simulink model "Model_TAGGED"  (R2022b)
settings: Solver=FixedStepDiscrete  StartTime=0.0  StopTime=100  RelTol=1e-3  EnableMultiTasking=on
InitFcn:
  | % Initialize model
  | ModelSettings=BTConfig.GetModelSettings();
  | 
  | ModelSettings.Validate();
  | 
  | ModelInit;
  | 
  | 
  | % load library data
  | GainLibrary_data;
StartFcn:
  | % make sure all the simulated RTC requests are found
  | %RTC_SIM_OBJ.ValidateREQs();
undefined symbols (not defined in the file or in its folder): MedusaConfig, sys_defs
libraries: FeaturePath x17, RTC x8, SampleRateConverterBtc x4, dspindex x3, EdgePorts x2, medusa5h1_stereo x2, FadeRamper x2, MuteRamper x2, SleepingBeauty x2, ToneBtc x2, dspsrcs4 x2, RouterBtc x1
(part 1 of 2)
settings Model: Creator=kl13806  LastModifiedBy=mp55777
settings SolverCC: AlgebraicLoopSolver=TrustRegion  AutoInsertRateTranBlk=on
settings OptimizationCC: DefaultParameterBehavior=Inlined  DefaultUnderspecifiedDataType=single  ZeroExternalMemoryAtStartup=off  ZeroInternalMemoryAtStartup=off  MaxStackSize=2048  DifferentSizesBufferReuse=on  EfficientTunableParamExpr=on
settings DebuggingCC: InheritedTsInSrcMsg=none  MultiTaskDSMMsg=none  MultiTaskRateTransMsg=warning  ParameterPrecisionLossMsg=none  ParameterTunabilityLossMsg=error  UnconnectedInputMsg=warning  UnconnectedOutputMsg=warning  UnconnectedLineMsg=warning  BusObjectLabelMismatch=none  UnknownTsInhSupMsg=none  SFUnexpectedBacktrackingDiag=warning  SFNoUnconditionalDefaultTransitionDiag=warning  SFExecutionAtInitializationDiag=none  SFMachineParentedDataDiag=warning  ArithmeticOperatorsInVariantConditions=warning
settings HardwareCC: ProdBitPerDouble=32  ProdBitPerPointer=32  ProdBitPerSizeT=32  ProdBitPerPtrDiffT=32  ProdLargestAtomicInteger=Long  ProdLargestAtomicFloat=Double  ProdWordSize=32  ProdHWDeviceType=Qualcomm->Hexagon  TargetBitPerPointer=64  TargetBitPerSizeT=64  TargetBitPerPtrDiffT=64  TargetLargestAtomicInteger=Integer  TargetLongLongMode=on  TargetIntDivRoundTo=Zero  TargetEndianess=LittleEndian  TargetWordSize=64  TargetHWDeviceType=MATLAB Host  ProdEqTarget=off
settings ModelReferenceCC: EnableRefExpFcnMdlSchedulingChecks=on
settings SFSimCC: SimUseLocalCustomCode=off  MATLABDynamicMemAlloc=off  CustomCodeUndefinedFunction=UseInterfaceOnly
settings RTWCC: Description=Embedded Coder (host-based shared library target)  SystemTargetFile=ert_shrlib.tlc  GenCodeOnly=on  TemplateMakefile=ert_default_tmf  GenerateReport=on  RetainRTWFile=on  RTWUseLocalCustomCode=off  BuildConfiguration=Faster Runs  IncludeHyperlinkInReport=on  GenerateTraceInfo=on  GenerateTraceReport=on  GenerateTraceReportSl=on  GenerateTraceReportSf=on  GenerateTraceReportEml=on  GenerateCodeMetricsReport=on  GenerateCodeReplacementReport=on
settings CodeAppCC: ForceParamTrailComments=on  IgnoreCustomStorageClasses=off  MaxIdLength=61  OperatorAnnotations=on  SimulinkDataObjDesc=on  SFDataObjDesc=on  MATLABFcnDesc=on  InsertBlockDesc=on  StateflowObjectComments=on  MATLABSourceComments=on
settings STFCustomTargetCC: TargetLangStandard=C99 (ISO)  CodeReplacementLibrary=Qualcomm Hexagon DSP code replacement library,ARM Neon V7/V8 code replacement library  ParMdlRefBuildCompliant=on  CompOptLevelCompliant=on  CombineOutputUpdateFcns=on  ERTCustomFileBanners=on  SupportNonFinite=off  SupportContinuousTime=off  SupportNonInlinedSFcns=off  RemoveResetFunc=on  SupportVariableSizeSignals=on  MATLABClassNameForMDSCustomization=Simulink.SoftwareTarget.ERTCustomization  ModelStepFunctionPrototypeControlCompliant=on  UseToolchainInfoCompliant=on  SystemTargetFile=ert_shrlib.tlc
settings ERTTargetCC: TargetLangStandard=C99 (ISO)  CodeReplacementLibrary=Qualcomm Hexagon DSP code replacement library,ARM Neon V7/V8 code replacement library  MultiwordLength=2048  ConcurrentExecutionCompliant=off  SupportNonFinite=off  SupportVariableSizeSignals=on  CPPClassGenCompliant=off  InlinedParameterPlacement=NonHierarchical  ERTCustomFileTemplate=example_file_process.tlc  IndentStyle=Allman  IndentSize=4
settings ConfigComp: CovMetricSettings=dw  CovSaveCumulativeToWorkspaceVar=on  CovSaveSingleToWorkspaceVar=on  CovExternalEMLEnable=off

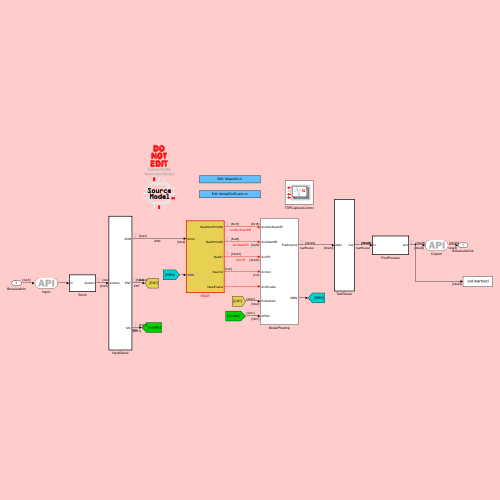
[thumbnail: Simulink's stored preview of the top-level diagram]
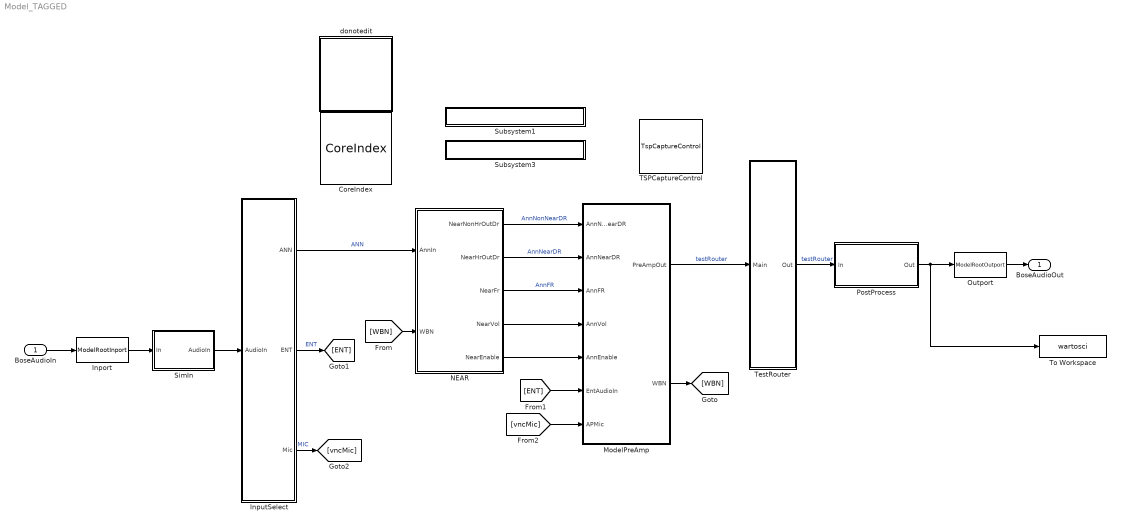
== system Model_TAGGED ==
  BoseAudioIn : Inport  OutDataTypeStr=single  PortDimensions=[ModelSettings.ModelFrameSize (ModelSettings.NumInputAudioChannels + ModelSettings.NumInputMicChannels)]  SampleTime=1/sys_defs.Fs * sys_defs.frameSize
  CoreIndex : FeaturePath/CoreIndex  Role=Source Model  CoreIndex=8  Config=[]  AddressingMode=Indirect core determination via table lookup (i.e. use Partition blocks)  CrossCoreApi=None  CrossCoreAllocation=None  CrossCoreSampleTime=-1  BasePeriod=[]  TriggerInit=[440 234 535 331]
      settings: SourceProductName=Bose Talaria
  Inport : EdgePorts/ModelRootInport  Config=ModelSettings.Inport
      settings: SourceProductName=Bose Talaria
  InputSelect : Subsystem  TreatAsAtomicUnit=on  mask{Config=ModelSettings.InputSelect}
      mask prompts: Config "InputSelectConfig"
      settings: RTWSystemCode=Nonreusable function
  ModelPreAmp : Subsystem  mask{Config=ModelSettings.ModelPreAmp}
      mask prompts: Config "PreAmpConfig"
  NEAR : Subsystem  TreatAsAtomicUnit=on  mask{Config=ModelSettings.NearConfig}
      mask prompts: Config "NearConfig"
  Outport : EdgePorts/ModelRootOutport  Config=ModelSettings.Outport
      settings: SourceProductName=Bose Talaria
  PostProcess : Subsystem  TreatAsAtomicUnit=on  mask{Config=ModelSettings.PostProcess}
      mask prompts: Config "PostProcessConfig"
  SimIn : Subsystem  TreatAsAtomicUnit=on
  Subsystem1 : Subsystem  mask{filename=Init.m}
      settings: OpenFcn=edit([ ModelRootName() get(gcbh,'filename') ]);
      mask Display: disp(['Edit: ' ModelRootName() get(gcbh,'filename')]);
  Subsystem3 : Subsystem  mask{filename=SimEvents.m}
      settings: OpenFcn=edit([ ModelRootName() get(gcbh,'filename') ]);
      mask Display: disp(['Edit: ' ModelRootName() get(gcbh,'filename')]);
  TSPCaptureControl : TSP/TspCaptureControl  TriggerInit=[870 244 955 316]
      settings: SourceProductName=Bose Talaria
  TestRouter : Subsystem  TreatAsAtomicUnit=on  mask{Config=ModelSettings.TestRouter}
      mask prompts: Config "TestRouterConfig"
  To Workspace : ToWorkspace  VariableName=wartosci  SaveFormat=Timeseries  SampleTime=-1
  donotedit : Subsystem
      settings: OpenFcn=Model
      mask Display: image('DoNotEdit.svg');
  BoseAudioOut : Outport  VectorParamsAs1DForOutWhenUnconnected=off
  wires:
  NEAR/3(NearFr) -> ModelPreAmp/3(AnnFR)  "AnnFR"
  NEAR/2(NearHrOutDr) -> ModelPreAmp/2(AnnNearDR)  "AnnNearDR"
  ModelPreAmp/1(PreAmpOut) -> TestRouter/1(Main)  "testRouter"
  NEAR/5(NearEnable) -> ModelPreAmp/5(AnnEnable)
  PostProcess/1(Out) -> To Workspace/1, Outport/1
  BoseAudioIn/1 -> Inport/1
  SimIn/1(AudioIn) -> InputSelect/1(AudioIn)
  Inport/1 -> SimIn/1(In)
  ModelPreAmp/2(WBN) -> [WBN]
  Outport/1 -> BoseAudioOut/1
  NEAR/4(NearVol) -> ModelPreAmp/4(AnnVol)
  [WBN] -> NEAR/2(WBN)
  InputSelect/1(ANN) -> NEAR/1(AnnIn)  "ANN"
  [vncMic] -> ModelPreAmp/7(APMic)
  InputSelect/2(ENT) -> [ENT]  "ENT"
  NEAR/1(NearNonHrOutDr) -> ModelPreAmp/1(AnnNonNearDR)  "AnnNonNearDR"
  InputSelect/3(Mic) -> [vncMic]  "MIC"
  [ENT] -> ModelPreAmp/6(EntAudioIn)
  TestRouter/1(Out) -> PostProcess/1(In)  "testRouter"

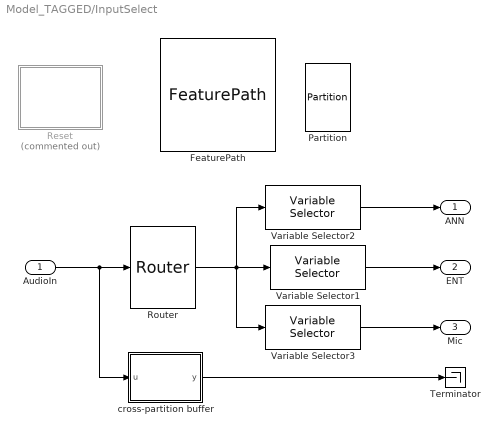
== system Model_TAGGED/InputSelect ==
  AudioIn : Inport
  FeaturePath : FeaturePath/FeaturePath  FeatureName=InputSelect  IsGroup=on  GroupNumber=0  IsModule=on  TriggerInit=[105 216 220 329]
      settings: SourceProductName=Bose Talaria
  Partition : FeaturePath/Partition  PartitionNumber=0  TriggerInit=[250 241 295 309]
      settings: SourceProductName=Bose Talaria
  Reset : Subsystem  Commented=on
  Router : RouterBtc/Router  Config=Config.RouterCfg  FeatureName=RouterCfg
      settings: SourceProductName=Bose Blocklib
  Terminator : Terminator
  Variable Selector1 : dspindex/Variable Selector  NumInputs=1  rowsOrCols=Columns  IdxMode=Fixed  Elements=Config.entMap  ZerOneIdxMode=One-based  errmode=Clip Index  FillMode=on  FillValues=0
  Variable Selector2 : dspindex/Variable Selector  NumInputs=1  rowsOrCols=Columns  IdxMode=Fixed  Elements=Config.annMap  ZerOneIdxMode=One-based  errmode=Clip Index  FillMode=on  FillValues=0
  Variable Selector3 : dspindex/Variable Selector  NumInputs=1  rowsOrCols=Columns  IdxMode=Fixed  Elements=Config.vncMic  ZerOneIdxMode=One-based  errmode=Clip Index  FillMode=on  FillValues=0
  cross-partition buffer : MATLAB Function  TreatAsAtomicUnit=on
  ANN : Outport
  ENT : Outport  Port=2  VectorParamsAs1DForOutWhenUnconnected=off
  Mic : Outport  Port=3
  wires:
  Variable Selector1/1 -> ENT/1
  AudioIn/1 -> cross-partition buffer/1(u), Router/1
  Router/1 -> Variable Selector2/1, Variable Selector3/1, Variable Selector1/1
  Variable Selector2/1 -> ANN/1
  Variable Selector3/1 -> Mic/1
  cross-partition buffer/1(y) -> Terminator/1

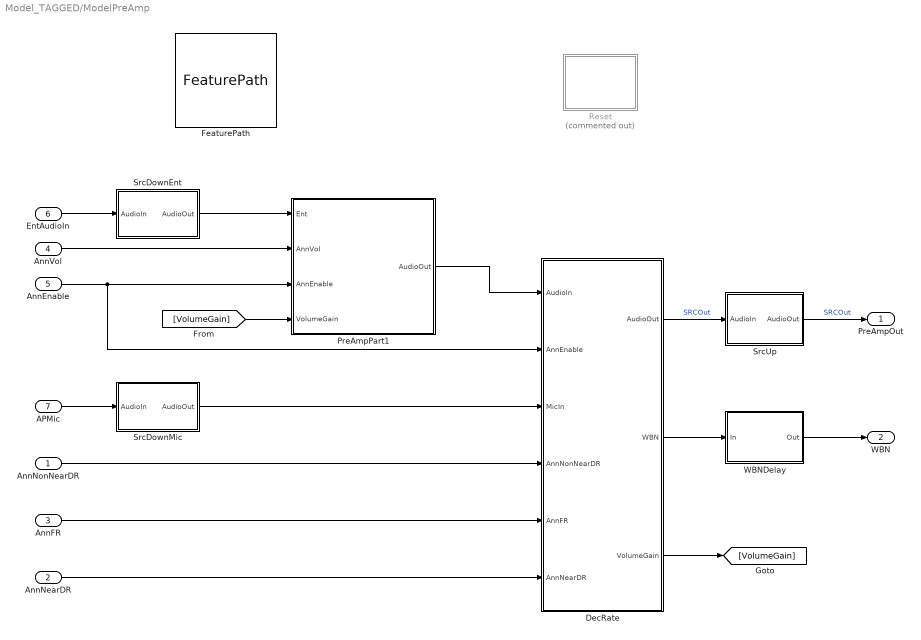
== system Model_TAGGED/ModelPreAmp ==
  AnnNonNearDR : Inport
  AnnNearDR : Inport  Port=2
  AnnFR : Inport  Port=3
  AnnVol : Inport  Port=4
  AnnEnable : Inport  Port=5
  EntAudioIn : Inport  Port=6
  APMic : Inport  Port=7
  DecRate : Subsystem
  FeaturePath : FeaturePath/FeaturePath  FeatureName=PreAmp  IsGroup=on  GroupNumber=2  IsModule=on  TriggerInit=[-135 -246 -20 -139]
      settings: SourceProductName=Bose Talaria
  PreAmpPart1 : Subsystem  TreatAsAtomicUnit=on
      settings: RTWSystemCode=Nonreusable function  FunctionWithSeparateData=on
  Reset : Subsystem  Commented=on  TreatAsAtomicUnit=on
  SrcDownEnt : Subsystem  TreatAsAtomicUnit=on
      settings: RTWSystemCode=Nonreusable function
  SrcDownMic : Subsystem  TreatAsAtomicUnit=on
      settings: RTWSystemCode=Nonreusable function
  SrcUp : Subsystem  TreatAsAtomicUnit=on
      settings: RTWSystemCode=Nonreusable function
  WBNDelay : Subsystem
  PreAmpOut : Outport  VectorParamsAs1DForOutWhenUnconnected=off
  WBN : Outport  Port=2
  wires:
  EntAudioIn/1 -> SrcDownEnt/1(AudioIn)
  DecRate/1(AudioOut) -> SrcUp/1(AudioIn)  "SRCOut"
  SrcUp/1(AudioOut) -> PreAmpOut/1  "SRCOut"
  SrcDownEnt/1(AudioOut) -> PreAmpPart1/1(Ent)
  AnnNonNearDR/1 -> DecRate/4(AnnNonNearDR)
  AnnNearDR/1 -> DecRate/6(AnnNearDR)
  AnnFR/1 -> DecRate/5(AnnFR)
  APMic/1 -> SrcDownMic/1(AudioIn)
  PreAmpPart1/1(AudioOut) -> DecRate/1(AudioIn)
  AnnEnable/1 -> DecRate/2(AnnEnable), PreAmpPart1/3(AnnEnable)
  SrcDownMic/1(AudioOut) -> DecRate/3(MicIn)
  DecRate/2(WBN) -> WBNDelay/1(In)
  WBNDelay/1(Out) -> WBN/1
  AnnVol/1 -> PreAmpPart1/2(AnnVol)
  DecRate/3(VolumeGain) -> [VolumeGain]
  [VolumeGain] -> PreAmpPart1/4(VolumeGain)

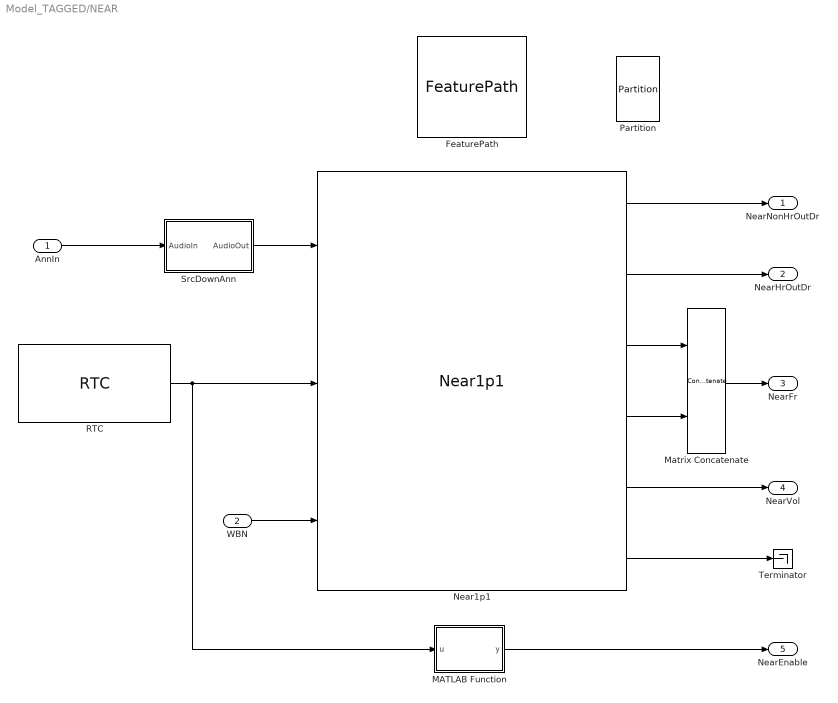
== system Model_TAGGED/NEAR ==
  AnnIn : Inport
  WBN : Inport  Port=2
  FeaturePath : FeaturePath/FeaturePath  FeatureName=Near  IsGroup=on  GroupNumber=1  IsModule=on  TriggerInit=[15 -306 130 -199]
      settings: SourceProductName=Bose Talaria
  MATLAB Function : MATLAB Function  TreatAsAtomicUnit=on
  Matrix Concatenate : Concatenate  Mode=Multidimensional array  ConcatenateDimension=2
  Near1p1 : Near1p1Ann/Near1p1  Config=Config.Near
  Partition : FeaturePath/Partition  PartitionNumber=0  TriggerInit=[225 -284 270 -216]
      settings: SourceProductName=Bose Talaria
  RTC : RTC/RTC  REQ_Priority=RTC_Mask.NormalPriority  RequestAtInit=off  EnableRequest=off  REQElemName1=Enable  REQElemType1=uint32  REQElemWidth1=1  REQElemInitial1=[0]  REQElemType2=uint32  REQElemWidth2=1  REQElemInitial2=[]  REQElemType3=uint32  REQElemWidth3=1  REQElemInitial3=[]  REQElemType4=uint32  REQElemWidth4=1  REQElemInitial4=[]  REQElemType5=uint32  REQElemWidth5=1  REQElemInitial5=[]  REQElemType6=uint32  REQElemWidth6=1  REQElemInitial6=[]  REQElemType7=uint32  REQElemWidth7=1  REQElemInitial7=[]  REQElemType8=uint32  REQElemWidth8=1  REQElemInitial8=[]  REQElemType9=uint32  REQElemWidth9=1  REQElemInitial9=[]  REQElemType10=uint32  REQElemWidth10=1  REQElemInitial10=[]  EnableResponse=on  EnableRSP_StatusIn=off  RSPElemType1=uint32  RSPElemWidth1=1  RSPElemType2=uint32  RSPElemWidth2=1  RSPElemType3=uint32  RSPElemWidth3=1  RSPElemType4=uint32  RSPElemWidth4=1  RSPElemType5=uint32  RSPElemWidth5=1  RSPElemType6=uint32  RSPElemWidth6=1  RSPElemType7=uint32  RSPElemWidth7=1  RSPElemType8=uint32  RSPElemWidth8=1  RSPElemType9=uint32  RSPElemWidth9=1  RSPElemType10=uint32  RSPElemWidth10=1  EnableNotification=off  EnableNTF_PrepTrig=off  NTFElemType1=uint32  NTFElemWidth1=1  NTFElemType2=uint32  NTFElemWidth2=1  NTFElemType3=uint32  NTFElemWidth3=1  NTFElemType4=uint32  NTFElemWidth4=1  NTFElemType5=uint32  NTFElemWidth5=1  NTFElemType6=uint32  NTFElemWidth6=1  NTFElemType7=uint32  NTFElemWidth7=1  NTFElemType8=uint32  NTFElemWidth8=1  NTFElemType9=uint32  NTFElemWidth9=1  NTFElemType10=uint32  NTFElemWidth10=1  MaskMessageName=Enable
      settings: SourceProductName=Bose Talaria
  SrcDownAnn : Subsystem  TreatAsAtomicUnit=on
      settings: RTWSystemCode=Nonreusable function
  Terminator : Terminator
  NearNonHrOutDr : Outport
  NearHrOutDr : Outport  Port=2
  NearFr : Outport  Port=3
  NearVol : Outport  Port=4
  NearEnable : Outport  Port=5
  wires:
  Near1p1/1 -> NearNonHrOutDr/1
  AnnIn/1 -> SrcDownAnn/1(AudioIn)
  Near1p1/2 -> NearHrOutDr/1
  Near1p1/3 -> Matrix Concatenate/1
  Near1p1/4 -> Matrix Concatenate/2
  Matrix Concatenate/1 -> NearFr/1
  Near1p1/5 -> NearVol/1
  Near1p1/6 -> Terminator/1
  RTC/1 -> MATLAB Function/1(u), Near1p1/2
  MATLAB Function/1(y) -> NearEnable/1
  SrcDownAnn/1(AudioOut) -> Near1p1/1
  WBN/1 -> Near1p1/3

== system Model_TAGGED/PostProcess ==
  In : Inport
  FeaturePath : FeaturePath/FeaturePath  FeatureName=PostProcess  IsGroup=on  GroupNumber=3  IsModule=on  TriggerInit=[85 -186 200 -79]
      settings: SourceProductName=Bose Talaria
  Partition : FeaturePath/Partition  PartitionNumber=0  TriggerInit=[225 -164 270 -96]
      settings: SourceProductName=Bose Talaria
  PostProcess : Subsystem  TreatAsAtomicUnit=on
      settings: RTWSystemCode=Nonreusable function  RTWFcnNameOpts=Use subsystem name  RTWFileNameOpts=Use subsystem name  FunctionWithSeparateData=on
  Reset : Subsystem  Commented=on
  Out : Outport  VectorParamsAs1DForOutWhenUnconnected=off
  wires:
  In/1 -> PostProcess/1(In)
  PostProcess/1(AudioOut) -> Out/1

== system Model_TAGGED/SimIn ==
  In : Inport  OutDataTypeStr=single  SampleTime=1/sys_defs.Fs * sys_defs.frameSize
  Colored Noise : dspsrcs4/Colored Noise  Commented=on  Color=pink  InverseFrequencyPower=1  BoundedOutput=on  NumChannels=2  OutputDataType=single  SamplesPerFrame=32  SampleTime=1/48000  RandomStream=mt19937ar with seed  Seed=67  SimulateUsing=Interpreted execution
  Sine Wave : dspsrcs4/Sine Wave  Amplitude=[ModelSettings.InputAudioChannelAmps ModelSettings.InputMicChannelAmps]  Frequency=[ModelSettings.InputAudioChannelFreqs ModelSettings.InputMicChannelFreqs]  Phase=zeros(1, numel([ModelSettings.InputAudioChannelFreqs ModelSettings.InputMicChannelFreqs]))  SampleMode=Discrete  OutComplex=Real  CompMethod=Trigonometric fcn  TableSize=Speed  SampleTime=1/ModelSettings.SampleRate  SamplesPerFrame=ModelSettings.ModelFrameSize  ResetState=Restart at time zero  OutputFrames=off  dataType=single  wordLen=16  udDataType=sfix(16)  fracBitsMode=Best precision  numFracBits=15  OutDataTypeStr=single  LastOutDataTypeStr=single
  Variant Source : VariantSource  VariantControlMode=sim codegen switching  ShowConditionOnBlock=on
  AudioIn : Outport  VectorParamsAs1DForOutWhenUnconnected=off
  wires:
  In/1 -> Variant Source/2
  Variant Source/1 -> AudioIn/1
  Sine Wave/1 -> Variant Source/1

== system Model_TAGGED/Subsystem1 ==

== system Model_TAGGED/Subsystem3 ==

== system Model_TAGGED/TestRouter ==
  Main : Inport
  ASDRouter : ASDRouter/ASDRouter  frameSize=Config.FrameSize  nChanOut=Config.NumChanOut  mainSelect=Config.MainSelect  numMainCh=Config.NumMainCh  mainGain=Config.MainGain  enableAux=Config.EnableAux  numAux=Config.NumAux  auxGain=Config.AuxGain
  FeaturePath : FeaturePath/FeaturePath  FeatureName=TestRouter  IsGroup=on  GroupNumber=5  IsModule=off  TriggerInit=[290 -166 405 -59]
      settings: SourceProductName=Bose Talaria
  Ground : Ground
  Matrix Concatenate : Concatenate  Mode=Multidimensional array  ConcatenateDimension=2
  Partition : FeaturePath/Partition  PartitionNumber=0  TriggerInit=[470 -149 515 -81]
      settings: SourceProductName=Bose Talaria
  TuneTOP : TuneVar/TuneTOP  TriggerInit=[175 117 345 173]  TopName=AuxSelect  TuneName=AuxSelect  DataTypeOut=int32  TunabilityNumber=1  MinValue=[]  MaxValue=[]  BankNumber=0  PreOverlay=false  PostOverlay=false  UseSameName=on  MaskValue=Config.MainGain
      settings: SourceProductName=Bose Talaria
  Out : Outport
  wires:
  ASDRouter/1 -> Out/1
  TuneTOP/1 -> ASDRouter/2
  Matrix Concatenate/1 -> ASDRouter/1
  Main/1 -> Matrix Concatenate/1
  Ground/1 -> Matrix Concatenate/2

== system Model_TAGGED/donotedit ==

== system Model_TAGGED/InputSelect/Reset ==
  MATLAB Function : MATLAB Function  TreatAsAtomicUnit=on
  RTC : RTC/RTC  REQ_Priority=RTC_Mask.NormalPriority  RequestAtInit=off  EnableRequest=on  REQElemType1=uint32  REQElemWidth1=1  REQElemInitial1=[]  REQElemType2=uint32  REQElemWidth2=1  REQElemInitial2=[]  REQElemType3=uint32  REQElemWidth3=1  REQElemInitial3=[]  REQElemType4=uint32  REQElemWidth4=1  REQElemInitial4=[]  REQElemType5=uint32  REQElemWidth5=1  REQElemInitial5=[]  REQElemType6=uint32  REQElemWidth6=1  REQElemInitial6=[]  REQElemType7=uint32  REQElemWidth7=1  REQElemInitial7=[]  REQElemType8=uint32  REQElemWidth8=1  REQElemInitial8=[]  REQElemType9=uint32  REQElemWidth9=1  REQElemInitial9=[]  REQElemType10=uint32  REQElemWidth10=1  REQElemInitial10=[]  EnableResponse=on  EnableRSP_StatusIn=off  RSPElemType1=uint32  RSPElemWidth1=1  RSPElemType2=uint32  RSPElemWidth2=1  RSPElemType3=uint32  RSPElemWidth3=1  RSPElemType4=uint32  RSPElemWidth4=1  RSPElemType5=uint32  RSPElemWidth5=1  RSPElemType6=uint32  RSPElemWidth6=1  RSPElemType7=uint32  RSPElemWidth7=1  RSPElemType8=uint32  RSPElemWidth8=1  RSPElemType9=uint32  RSPElemWidth9=1  RSPElemType10=uint32  RSPElemWidth10=1  EnableNotification=off  EnableNTF_PrepTrig=off  NTFElemType1=uint32  NTFElemWidth1=1  NTFElemType2=uint32  NTFElemWidth2=1  NTFElemType3=uint32  NTFElemWidth3=1  NTFElemType4=uint32  NTFElemWidth4=1  NTFElemType5=uint32  NTFElemWidth5=1  NTFElemType6=uint32  NTFElemWidth6=1  NTFElemType7=uint32  NTFElemWidth7=1  NTFElemType8=uint32  NTFElemWidth8=1  NTFElemType9=uint32  NTFElemWidth9=1  NTFElemType10=uint32  NTFElemWidth10=1  MaskMessageName=Reset
      settings: SourceProductName=Bose Talaria
  wires:
  RTC/1 -> MATLAB Function/Trigger

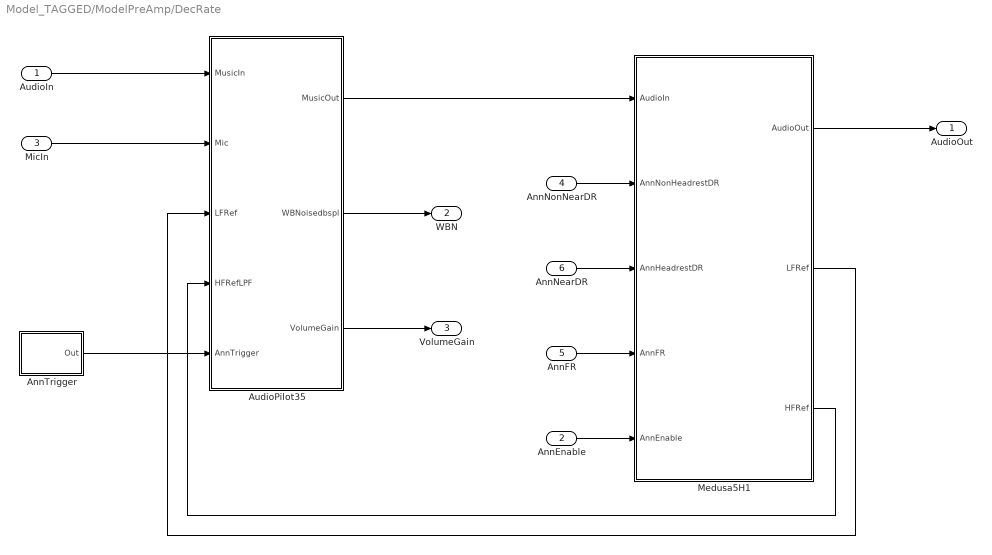
== system Model_TAGGED/ModelPreAmp/DecRate ==
  AudioIn : Inport
  AnnEnable : Inport  Port=2
  MicIn : Inport  Port=3
  AnnNonNearDR : Inport  Port=4
  AnnFR : Inport  Port=5
  AnnNearDR : Inport  Port=6
  AnnTrigger : Subsystem  TreatAsAtomicUnit=on
  AudioPilot35 : Subsystem  TreatAsAtomicUnit=on
      settings: RTWFcnNameOpts=Use subsystem name  RTWFileNameOpts=Use subsystem name  FunctionWithSeparateData=on
  Medusa5H1 : Subsystem
  AudioOut : Outport
  WBN : Outport  Port=2
  VolumeGain : Outport  Port=3
  wires:
  Medusa5H1/1(AudioOut) -> AudioOut/1
  MicIn/1 -> AudioPilot35/2(Mic)
  Medusa5H1/2(LFRef) -> AudioPilot35/3(LFRef)
  Medusa5H1/3(HFRef) -> AudioPilot35/4(HFRefLPF)
  AnnEnable/1 -> Medusa5H1/5(AnnEnable)
  AnnNonNearDR/1 -> Medusa5H1/2(AnnNonHeadrestDR)
  AnnNearDR/1 -> Medusa5H1/3(AnnHeadrestDR)
  AnnFR/1 -> Medusa5H1/4(AnnFR)
  AudioIn/1 -> AudioPilot35/1(MusicIn)
  AudioPilot35/1(MusicOut) -> Medusa5H1/1(AudioIn)
  AudioPilot35/2(WBNoisedbspl) -> WBN/1
  AnnTrigger/1(Out) -> AudioPilot35/5(AnnTrigger)
  AudioPilot35/3(VolumeGain) -> VolumeGain/1

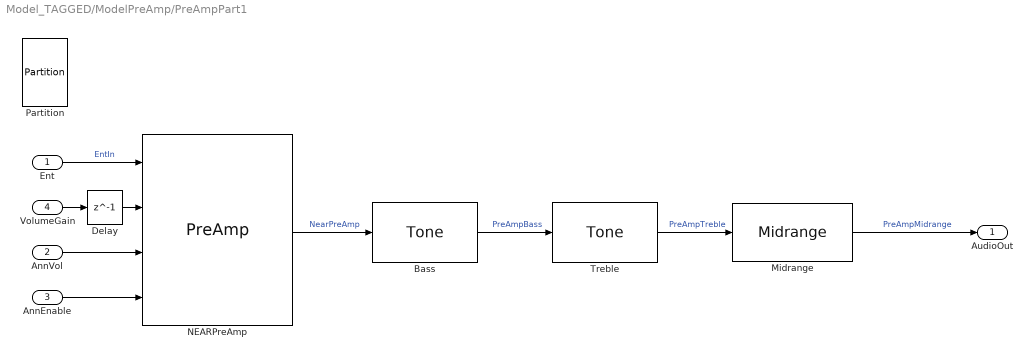
== system Model_TAGGED/ModelPreAmp/PreAmpPart1 ==
  Ent : Inport
  AnnVol : Inport  Port=2
  AnnEnable : Inport  Port=3
  VolumeGain : Inport  Port=4
  Bass : ToneBtc/Tone  FeatureName=Bass  Config=Config.Bass  TriggerInit=[215 80 320 140]
      settings: SourceProductName=Bose Blocklib
  Delay : Delay  DelayLength=1
  Midrange : MidrangeBtc/Midrange  FeatureName=Midrange  Config=Config.Midrange
      settings: SourceProductName=Bose Blocklib
  NEARPreAmp : PreAmpLib/PreAmp  Config=Config.NearPreAmpConfig
  Partition : FeaturePath/Partition  PartitionNumber=0  TriggerInit=[-135 -84 -90 -16]
      settings: SourceProductName=Bose Talaria
  Treble : ToneBtc/Tone  FeatureName=Treble  Config=Config.Treble  TriggerInit=[395 80 500 140]
      settings: SourceProductName=Bose Blocklib
  AudioOut : Outport
  wires:
  Ent/1 -> NEARPreAmp/1  "EntIn"
  Bass/1 -> Treble/1  "PreAmpBass"
  Treble/1 -> Midrange/1  "PreAmpTreble"
  Midrange/1 -> AudioOut/1  "PreAmpMidrange"
  NEARPreAmp/1 -> Bass/1  "NearPreAmp"
  AnnVol/1 -> NEARPreAmp/3
  AnnEnable/1 -> NEARPreAmp/4
  Delay/1 -> NEARPreAmp/2
  VolumeGain/1 -> Delay/1

== system Model_TAGGED/ModelPreAmp/Reset ==
  MATLAB Function : MATLAB Function  TreatAsAtomicUnit=on
  Partition : FeaturePath/Partition  PartitionNumber=12  TriggerInit=[245 -74 290 -6]
      settings: SourceProductName=Bose Talaria
  RTC : RTC/RTC  REQ_Priority=RTC_Mask.NormalPriority  RequestAtInit=off  EnableRequest=on  REQElemType1=uint32  REQElemWidth1=1  REQElemInitial1=[]  REQElemType2=uint32  REQElemWidth2=1  REQElemInitial2=[]  REQElemType3=uint32  REQElemWidth3=1  REQElemInitial3=[]  REQElemType4=uint32  REQElemWidth4=1  REQElemInitial4=[]  REQElemType5=uint32  REQElemWidth5=1  REQElemInitial5=[]  REQElemType6=uint32  REQElemWidth6=1  REQElemInitial6=[]  REQElemType7=uint32  REQElemWidth7=1  REQElemInitial7=[]  REQElemType8=uint32  REQElemWidth8=1  REQElemInitial8=[]  REQElemType9=uint32  REQElemWidth9=1  REQElemInitial9=[]  REQElemType10=uint32  REQElemWidth10=1  REQElemInitial10=[]  EnableResponse=on  EnableRSP_StatusIn=off  RSPElemType1=uint32  RSPElemWidth1=1  RSPElemType2=uint32  RSPElemWidth2=1  RSPElemType3=uint32  RSPElemWidth3=1  RSPElemType4=uint32  RSPElemWidth4=1  RSPElemType5=uint32  RSPElemWidth5=1  RSPElemType6=uint32  RSPElemWidth6=1  RSPElemType7=uint32  RSPElemWidth7=1  RSPElemType8=uint32  RSPElemWidth8=1  RSPElemType9=uint32  RSPElemWidth9=1  RSPElemType10=uint32  RSPElemWidth10=1  EnableNotification=off  EnableNTF_PrepTrig=off  NTFElemType1=uint32  NTFElemWidth1=1  NTFElemType2=uint32  NTFElemWidth2=1  NTFElemType3=uint32  NTFElemWidth3=1  NTFElemType4=uint32  NTFElemWidth4=1  NTFElemType5=uint32  NTFElemWidth5=1  NTFElemType6=uint32  NTFElemWidth6=1  NTFElemType7=uint32  NTFElemWidth7=1  NTFElemType8=uint32  NTFElemWidth8=1  NTFElemType9=uint32  NTFElemWidth9=1  NTFElemType10=uint32  NTFElemWidth10=1  MaskMessageName=Reset
      settings: SourceProductName=Bose Talaria
  wires:
  RTC/1 -> MATLAB Function/Trigger

== system Model_TAGGED/ModelPreAmp/SrcDownEnt ==
  AudioIn : Inport
  Frame Conversion1 : FrameConversion  OutFrame=Sample-based
  Frame Conversion2 : FrameConversion
  src : SampleRateConverterBtc/SampleRateConverter  Config=Config.SrcDn
      settings: SourceProductName=Bose Blocklib
  AudioOut : Outport
  wires:
  src/1 -> Frame Conversion1/1
  AudioIn/1 -> Frame Conversion2/1
  Frame Conversion1/1 -> AudioOut/1
  Frame Conversion2/1 -> src/1

== system Model_TAGGED/ModelPreAmp/SrcDownMic ==
  AudioIn : Inport
  Frame Conversion1 : FrameConversion  OutFrame=Sample-based
  Frame Conversion2 : FrameConversion
  InnerLink : SampleRateConverterBtc/SampleRateConverter  Config=Config.SrcDn
      settings: SourceProductName=Bose Blocklib
  AudioOut : Outport
  wires:
  InnerLink/1 -> Frame Conversion1/1
  AudioIn/1 -> Frame Conversion2/1
  Frame Conversion1/1 -> AudioOut/1
  Frame Conversion2/1 -> InnerLink/1

== system Model_TAGGED/ModelPreAmp/SrcUp ==
  AudioIn : Inport
  Frame Conversion : FrameConversion
  Frame Conversion1 : FrameConversion  OutFrame=Sample-based
  src : SampleRateConverterBtc/SampleRateConverter  Config=Config.SrcUp
      settings: SourceProductName=Bose Blocklib
  AudioOut : Outport
  wires:
  src/1 -> Frame Conversion1/1
  Frame Conversion/1 -> src/1
  Frame Conversion1/1 -> AudioOut/1
  AudioIn/1 -> Frame Conversion/1

== system Model_TAGGED/ModelPreAmp/WBNDelay ==
  In : Inport
  Delay3 : Delay  DelayLength=1
  Out : Outport
  wires:
  Delay3/1 -> Out/1
  In/1 -> Delay3/1

== system Model_TAGGED/NEAR/SrcDownAnn ==
  AudioIn : Inport
  Frame Conversion1 : FrameConversion  OutFrame=Sample-based
  Frame Conversion2 : FrameConversion
  src : SampleRateConverterBtc/SampleRateConverter  Config=Config.SrcDn
      settings: SourceProductName=Bose Blocklib
  AudioOut : Outport
  wires:
  src/1 -> Frame Conversion1/1
  AudioIn/1 -> Frame Conversion2/1
  Frame Conversion1/1 -> AudioOut/1
  Frame Conversion2/1 -> src/1

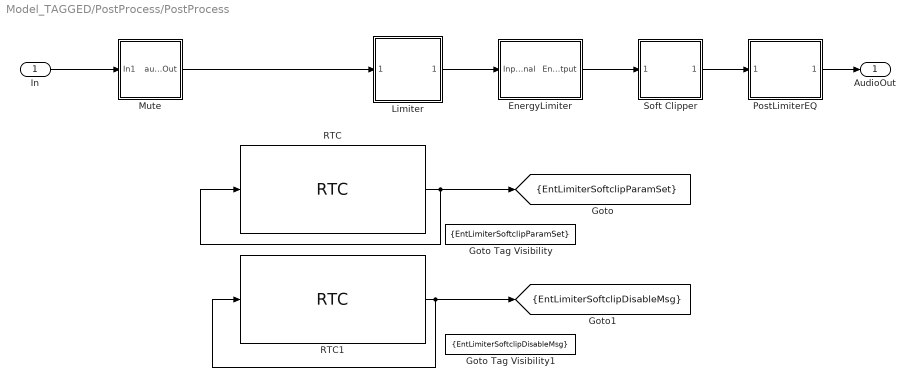
== system Model_TAGGED/PostProcess/PostProcess ==
  In : Inport
  EnergyLimiter : Subsystem
  Goto Tag Visibility : GotoTagVisibility  GotoTag=EntLimiterSoftclipParamSet
  Goto Tag Visibility1 : GotoTagVisibility  GotoTag=EntLimiterSoftclipDisableMsg
  Limiter : Subsystem
  Mute : Subsystem
  PostLimiterEQ : Subsystem
  RTC : RTC/RTC  Description=|  REQ_Priority=RTC_Mask.NormalPriority  RequestAtInit=off  EnableRequest=off  REQElemName1=paramSet  REQElemType1=uint32  REQElemWidth1=1  REQElemInitial1=1  REQElemType2=uint32  REQElemWidth2=1  REQElemInitial2=[]  REQElemType3=uint32  REQElemWidth3=1  REQElemInitial3=[]  REQElemType4=uint32  REQElemWidth4=1  REQElemInitial4=[]  REQElemType5=uint32  REQElemWidth5=1  REQElemInitial5=[]  REQElemType6=uint32  REQElemWidth6=1  REQElemInitial6=[]  REQElemType7=uint32  REQElemWidth7=1  REQElemInitial7=[]  REQElemType8=uint32  REQElemWidth8=1  REQElemInitial8=[]  REQElemType9=uint32  REQElemWidth9=1  REQElemInitial9=[]  REQElemType10=uint32  REQElemWidth10=1  REQElemInitial10=[]  EnableResponse=on  EnableRSP_StatusIn=off  RSPElemName1=paramSet  RSPElemType1=uint32  RSPElemWidth1=1  RSPElemType2=uint32  RSPElemWidth2=1  RSPElemType3=uint32  RSPElemWidth3=1  RSPElemType4=uint32  RSPElemWidth4=1  RSPElemType5=uint32  RSPElemWidth5=1  RSPElemType6=uint32  RSPElemWidth6=1  RSPElemType7=uint32  RSPElemWidth7=1  RSPElemType8=uint32  RSPElemWidth8=1  RSPElemType9=uint32  RSPElemWidth9=1  RSPElemType10=uint32  RSPElemWidth10=1  EnableNotification=off  EnableNTF_PrepTrig=off  NTFElemType1=uint32  NTFElemWidth1=1  NTFElemType2=uint32  NTFElemWidth2=1  NTFElemType3=uint32  NTFElemWidth3=1  NTFElemType4=uint32  NTFElemWidth4=1  NTFElemType5=uint32  NTFElemWidth5=1  NTFElemType6=uint32  NTFElemWidth6=1  NTFElemType7=uint32  NTFElemWidth7=1  NTFElemType8=uint32  NTFElemWidth8=1  NTFElemType9=uint32  NTFElemWidth9=1  NTFElemType10=uint32  NTFElemWidth10=1  MaskMessageName=LimiterSoftclipParamSet
      | Choose parameter set for limiter and soft clipper.
      | 1: normal set
      | 2: used in start-stop situation
      settings: SourceProductName=Bose Talaria
  RTC1 : RTC/RTC  REQ_Priority=RTC_Mask.NormalPriority  RequestAtInit=off  EnableRequest=off  REQElemName1=disableMsg  REQElemType1=uint32  REQElemWidth1=1  REQElemInitial1=0  REQElemType2=uint32  REQElemWidth2=1  REQElemInitial2=[]  REQElemType3=uint32  REQElemWidth3=1  REQElemInitial3=[]  REQElemType4=uint32  REQElemWidth4=1  REQElemInitial4=[]  REQElemType5=uint32  REQElemWidth5=1  REQElemInitial5=[]  REQElemType6=uint32  REQElemWidth6=1  REQElemInitial6=[]  REQElemType7=uint32  REQElemWidth7=1  REQElemInitial7=[]  REQElemType8=uint32  REQElemWidth8=1  REQElemInitial8=[]  REQElemType9=uint32  REQElemWidth9=1  REQElemInitial9=[]  REQElemType10=uint32  REQElemWidth10=1  REQElemInitial10=[]  EnableResponse=on  EnableRSP_StatusIn=off  RSPElemName1=disableMsg  RSPElemType1=uint32  RSPElemWidth1=1  RSPElemType2=uint32  RSPElemWidth2=1  RSPElemType3=uint32  RSPElemWidth3=1  RSPElemType4=uint32  RSPElemWidth4=1  RSPElemType5=uint32  RSPElemWidth5=1  RSPElemType6=uint32  RSPElemWidth6=1  RSPElemType7=uint32  RSPElemWidth7=1  RSPElemType8=uint32  RSPElemWidth8=1  RSPElemType9=uint32  RSPElemWidth9=1  RSPElemType10=uint32  RSPElemWidth10=1  EnableNotification=off  EnableNTF_PrepTrig=off  NTFElemType1=uint32  NTFElemWidth1=1  NTFElemType2=uint32  NTFElemWidth2=1  NTFElemType3=uint32  NTFElemWidth3=1  NTFElemType4=uint32  NTFElemWidth4=1  NTFElemType5=uint32  NTFElemWidth5=1  NTFElemType6=uint32  NTFElemWidth6=1  NTFElemType7=uint32  NTFElemWidth7=1  NTFElemType8=uint32  NTFElemWidth8=1  NTFElemType9=uint32  NTFElemWidth9=1  NTFElemType10=uint32  NTFElemWidth10=1  MaskMessageName=LimiterSoftclipDisable
      settings: SourceProductName=Bose Talaria
  Soft Clipper : Subsystem
  AudioOut : Outport  VectorParamsAs1DForOutWhenUnconnected=off
  tag scope: EntLimiterSoftclipDisableMsg=scoped, EntLimiterSoftclipParamSet=scoped
  wires:
  In/1 -> Mute/1(In1)
  EnergyLimiter/1(EnergyLimOutput) -> Soft Clipper/1(AudioIn)
  RTC1/1 -> RTC1/1, [EntLimiterSoftclipDisableMsg]
  RTC/1 -> RTC/1, [EntLimiterSoftclipParamSet]
  Soft Clipper/1(" AudioOut") -> PostLimiterEQ/1(AudioIn)
  Mute/1(audioOut) -> Limiter/1(AudioIn)
  Limiter/1(AudioOut) -> EnergyLimiter/1(InputSignal)
  PostLimiterEQ/1(AudioOut) -> AudioOut/1

== system Model_TAGGED/PostProcess/Reset ==
  MATLAB Function : MATLAB Function  TreatAsAtomicUnit=on
  RTC : RTC/RTC  REQ_Priority=RTC_Mask.NormalPriority  RequestAtInit=off  EnableRequest=on  REQElemType1=uint32  REQElemWidth1=1  REQElemInitial1=[]  REQElemType2=uint32  REQElemWidth2=1  REQElemInitial2=[]  REQElemType3=uint32  REQElemWidth3=1  REQElemInitial3=[]  REQElemType4=uint32  REQElemWidth4=1  REQElemInitial4=[]  REQElemType5=uint32  REQElemWidth5=1  REQElemInitial5=[]  REQElemType6=uint32  REQElemWidth6=1  REQElemInitial6=[]  REQElemType7=uint32  REQElemWidth7=1  REQElemInitial7=[]  REQElemType8=uint32  REQElemWidth8=1  REQElemInitial8=[]  REQElemType9=uint32  REQElemWidth9=1  REQElemInitial9=[]  REQElemType10=uint32  REQElemWidth10=1  REQElemInitial10=[]  EnableResponse=on  EnableRSP_StatusIn=off  RSPElemType1=uint32  RSPElemWidth1=1  RSPElemType2=uint32  RSPElemWidth2=1  RSPElemType3=uint32  RSPElemWidth3=1  RSPElemType4=uint32  RSPElemWidth4=1  RSPElemType5=uint32  RSPElemWidth5=1  RSPElemType6=uint32  RSPElemWidth6=1  RSPElemType7=uint32  RSPElemWidth7=1  RSPElemType8=uint32  RSPElemWidth8=1  RSPElemType9=uint32  RSPElemWidth9=1  RSPElemType10=uint32  RSPElemWidth10=1  EnableNotification=off  EnableNTF_PrepTrig=off  NTFElemType1=uint32  NTFElemWidth1=1  NTFElemType2=uint32  NTFElemWidth2=1  NTFElemType3=uint32  NTFElemWidth3=1  NTFElemType4=uint32  NTFElemWidth4=1  NTFElemType5=uint32  NTFElemWidth5=1  NTFElemType6=uint32  NTFElemWidth6=1  NTFElemType7=uint32  NTFElemWidth7=1  NTFElemType8=uint32  NTFElemWidth8=1  NTFElemType9=uint32  NTFElemWidth9=1  NTFElemType10=uint32  NTFElemWidth10=1  MaskMessageName=Reset
      settings: SourceProductName=Bose Talaria
  wires:
  RTC/1 -> MATLAB Function/Trigger

== system Model_TAGGED/ModelPreAmp/DecRate/AnnTrigger ==
  Constant : Constant  Value=0  SampleTime=-1
  Out : Outport
  wires:
  Constant/1 -> Out/1

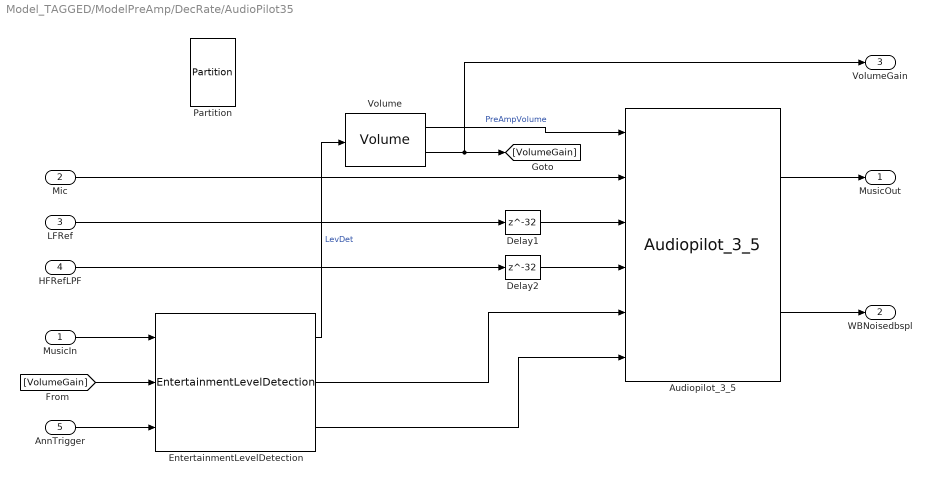
== system Model_TAGGED/ModelPreAmp/DecRate/AudioPilot35 ==
  MusicIn : Inport
  Mic : Inport  Port=2
  LFRef : Inport  Port=3
  HFRefLPF : Inport  Port=4
  AnnTrigger : Inport  Port=5
  Audiopilot_3_5 : Audiopilot_3_5/Audiopilot_3_5  FeatureName=Audiopilot  InputAudioMode=Stereo - 2 Channels  NoiseEstimationMode=Regular  IncludeSpumTails=off  IncludeIgnoreMicFlag=off  Config=Config.Audiopilot
  Delay1 : Delay  DelayLength=32
  Delay2 : Delay  DelayLength=32
  EntertainmentLevelDetection : EntertainmentLevelDetection/EntertainmentLevelDetection  NumInputChannels=Config.AudiopilotNumMusicIn  FANEnable=off  BODEnable=off  Config=Config.LDCfg
  Partition : FeaturePath/Partition  PartitionNumber=4  TriggerInit=[-55 -104 -10 -36]
      settings: SourceProductName=Bose Talaria
  Volume : VolumeBtc/Volume  FeatureName=VolumeCfg  Config=Config.VolumeCfg  EnableGainOut=on  TriggerInit=[100 -29 180 24]
      settings: SourceProductName=Bose Blocklib
  MusicOut : Outport
  WBNoisedbspl : Outport  Port=2
  VolumeGain : Outport  Port=3
  wires:
  MusicIn/1 -> EntertainmentLevelDetection/1
  AnnTrigger/1 -> EntertainmentLevelDetection/3
  EntertainmentLevelDetection/1 -> Volume/1  "LevDet"
  LFRef/1 -> Delay1/1
  Audiopilot_3_5/2 -> WBNoisedbspl/1
  HFRefLPF/1 -> Delay2/1
  Audiopilot_3_5/1 -> MusicOut/1
  EntertainmentLevelDetection/2 -> Audiopilot_3_5/5
  EntertainmentLevelDetection/3 -> Audiopilot_3_5/6
  Mic/1 -> Audiopilot_3_5/2
  Delay1/1 -> Audiopilot_3_5/3
  Delay2/1 -> Audiopilot_3_5/4
  Volume/1 -> Audiopilot_3_5/1  "PreAmpVolume"
  Volume/2 -> VolumeGain/1, [VolumeGain]
  [VolumeGain] -> EntertainmentLevelDetection/2

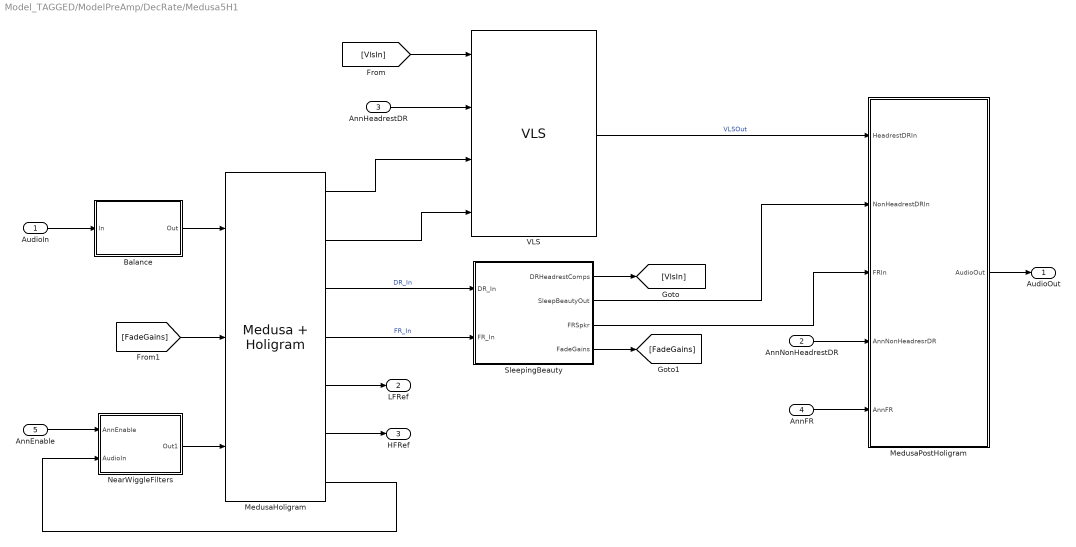
== system Model_TAGGED/ModelPreAmp/DecRate/Medusa5H1 ==
  AudioIn : Inport
  AnnNonHeadrestDR : Inport  Port=2
  AnnHeadrestDR : Inport  Port=3
  AnnFR : Inport  Port=4
  AnnEnable : Inport  Port=5
  Balance : Subsystem  TreatAsAtomicUnit=on
  MedusaHoligram : medusa5h1_stereo/Medusa + Holigram  config=Config.MedusaConfig  ConfigBTC=Config.MedusaBTC  vlsConfigStruct=Config.VLSConfig
      link override Medusa5H1 Part 1/Bass Manager Stereo/Variant Subsystem/Discrete: VariantControl=(ConfigBTC.BassManager.NumInputs > 2)
      link override Medusa5H1 Part 1/Bass Manager Stereo/Variant Subsystem/Stereo: VariantControl=(ConfigBTC.BassManager.NumInputs == 2)
      link override Medusa5H1 Part 2/Decimated-Rate FDP/Fdp/FreqDomainProcessing/CalculateAndApplyCoefficients/DeciRate: VariantControl="Config.Variant == \"DeciRate\""
      link override Medusa5H1 Part 2/Decimated-Rate FDP/Fdp/FreqDomainProcessing/CalculateAndApplyCoefficients/FullRate: VariantControl="Config.Variant == \"FullRate\""
  MedusaPostHoligram : Subsystem  TreatAsAtomicUnit=on
  NearWiggleFilters : Subsystem  TreatAsAtomicUnit=on
  SleepingBeauty : Subsystem  TreatAsAtomicUnit=on
  VLS : VLS/VLS  configStruct=Config.VLSConfig
      link override Partition: PartitionNumber=10
  AudioOut : Outport
  LFRef : Outport  Port=2
  HFRef : Outport  Port=3
  wires:
  MedusaHoligram/6 -> HFRef/1
  MedusaHoligram/2 -> VLS/4
  MedusaHoligram/1 -> VLS/3
  MedusaHoligram/5 -> LFRef/1
  AudioIn/1 -> Balance/1(In)
  Balance/1(Out) -> MedusaHoligram/1
  AnnHeadrestDR/1 -> VLS/2
  AnnNonHeadrestDR/1 -> MedusaPostHoligram/4(AnnNonHeadresrDR)
  AnnFR/1 -> MedusaPostHoligram/5(AnnFR)
  VLS/1 -> MedusaPostHoligram/1(HeadrestDRIn)  "VLSOut"
  MedusaPostHoligram/1(AudioOut) -> AudioOut/1
  [VlsIn] -> VLS/1
  AnnEnable/1 -> NearWiggleFilters/1(AnnEnable)
  [FadeGains] -> MedusaHoligram/2
  NearWiggleFilters/1(Out1) -> MedusaHoligram/3
  MedusaHoligram/7 -> NearWiggleFilters/2(AudioIn)
  MedusaHoligram/3 -> SleepingBeauty/1(DR_In)  "DR_In"
  MedusaHoligram/4 -> SleepingBeauty/2(FR_In)  "FR_In"
  SleepingBeauty/1(DRHeadrestComps) -> [VlsIn]
  SleepingBeauty/2(SleepBeautyOut) -> MedusaPostHoligram/2(NonHeadrestDRIn)
  SleepingBeauty/3(FRSpkr) -> MedusaPostHoligram/3(FRIn)
  SleepingBeauty/4(FadeGains) -> [FadeGains]

== system Model_TAGGED/PostProcess/PostProcess/EnergyLimiter ==
  InputSignal : Inport
  EnergyLimiter1 : EnergyLimiterBtc/EnergyLimiter  Config=Config.EnergyLimiter  FeatureName=EnergyLimiter
      link override EnergyRunningAvg /Alpha/ConstantFrameSize: Value=- Config.FrameSize
      settings: SourceProductName=Bose Blocklib
  Terminator : Terminator
  EnergyLimOutput : Outport
  wires:
  EnergyLimiter1/2 -> Terminator/1
  InputSignal/1 -> EnergyLimiter1/1
  EnergyLimiter1/1 -> EnergyLimOutput/1

== system Model_TAGGED/PostProcess/PostProcess/Limiter ==
  AudioIn : Inport
  Limiter : LimiterBtc/Limiter  Config=Config.Limiter  FeatureName=Limiter
      settings: SourceProductName=Bose Blocklib
  Terminator : Terminator
  AudioOut : Outport  VectorParamsAs1DForOutWhenUnconnected=off
  wires:
  AudioIn/1 -> Limiter/1
  Limiter/1 -> AudioOut/1
  [EntLimiterSoftclipParamSet] -> Limiter/2
  [EntLimiterSoftclipDisableMsg] -> Limiter/3
  Limiter/2 -> Terminator/1

== system Model_TAGGED/PostProcess/PostProcess/Mute ==
  In1 : Inport
  Mute : MuteBtc/Mute  Config=Config.Mute  FeatureName=Mute
      settings: SourceProductName=Bose Blocklib
  audioOut : Outport  VectorParamsAs1DForOutWhenUnconnected=off
  wires:
  In1/1 -> Mute/1
  Mute/1 -> audioOut/1

== system Model_TAGGED/PostProcess/PostProcess/PostLimiterEQ ==
  AudioIn : Inport
  PoolIirTunableWithReset : PoolIir/PoolIirTunableWithReset  FeatureName=PostLimiterEq  Config=Config.PostLimiterEq
      settings: SourceProductName=Bose Blocklib
  RTC : RTC/RTC  REQ_Priority=RTC_Mask.NormalPriority  RequestAtInit=off  EnableRequest=on  REQElemType1=uint32  REQElemWidth1=1  REQElemInitial1=[]  REQElemType2=uint32  REQElemWidth2=1  REQElemInitial2=[]  REQElemType3=uint32  REQElemWidth3=1  REQElemInitial3=[]  REQElemType4=uint32  REQElemWidth4=1  REQElemInitial4=[]  REQElemType5=uint32  REQElemWidth5=1  REQElemInitial5=[]  REQElemType6=uint32  REQElemWidth6=1  REQElemInitial6=[]  REQElemType7=uint32  REQElemWidth7=1  REQElemInitial7=[]  REQElemType8=uint32  REQElemWidth8=1  REQElemInitial8=[]  REQElemType9=uint32  REQElemWidth9=1  REQElemInitial9=[]  REQElemType10=uint32  REQElemWidth10=1  REQElemInitial10=[]  EnableResponse=on  EnableRSP_StatusIn=off  RSPElemType1=uint32  RSPElemWidth1=1  RSPElemType2=uint32  RSPElemWidth2=1  RSPElemType3=uint32  RSPElemWidth3=1  RSPElemType4=uint32  RSPElemWidth4=1  RSPElemType5=uint32  RSPElemWidth5=1  RSPElemType6=uint32  RSPElemWidth6=1  RSPElemType7=uint32  RSPElemWidth7=1  RSPElemType8=uint32  RSPElemWidth8=1  RSPElemType9=uint32  RSPElemWidth9=1  RSPElemType10=uint32  RSPElemWidth10=1  EnableNotification=off  EnableNTF_PrepTrig=off  NTFElemType1=uint32  NTFElemWidth1=1  NTFElemType2=uint32  NTFElemWidth2=1  NTFElemType3=uint32  NTFElemWidth3=1  NTFElemType4=uint32  NTFElemWidth4=1  NTFElemType5=uint32  NTFElemWidth5=1  NTFElemType6=uint32  NTFElemWidth6=1  NTFElemType7=uint32  NTFElemWidth7=1  NTFElemType8=uint32  NTFElemWidth8=1  NTFElemType9=uint32  NTFElemWidth9=1  NTFElemType10=uint32  NTFElemWidth10=1  MaskMessageName=PostLimiterEqShutdown
      settings: SourceProductName=Bose Talaria
  AudioOut : Outport
  wires:
  AudioIn/1 -> PoolIirTunableWithReset/1
  RTC/1 -> PoolIirTunableWithReset/2
  PoolIirTunableWithReset/1 -> AudioOut/1

== system Model_TAGGED/PostProcess/PostProcess/Soft Clipper ==
  AudioIn : Inport
  SoftClipper : SoftclipperBtc/SoftClipper  Config=Config.SoftClipper  FeatureName=SoftClipper
      settings: SourceProductName=Bose Blocklib
  Terminator : Terminator
  " AudioOut" : Outport  VectorParamsAs1DForOutWhenUnconnected=off
  wires:
  AudioIn/1 -> SoftClipper/1
  SoftClipper/1 -> " AudioOut"/1
  [EntLimiterSoftclipParamSet] -> SoftClipper/2
  [EntLimiterSoftclipDisableMsg] -> SoftClipper/3
  SoftClipper/2 -> Terminator/1

== system Model_TAGGED/ModelPreAmp/DecRate/Medusa5H1/Balance ==
  In : Inport
  Balance : BalanceBtc/Balance  FeatureName=Balance_Cfg  Config=Config.Balance_Cfg
      settings: SourceProductName=Bose Blocklib
  Partition : FeaturePath/Partition  PartitionNumber=11  TriggerInit=[325 -4 370 64]
      settings: SourceProductName=Bose Talaria
  Out : Outport
  wires:
  Balance/1 -> Out/1
  In/1 -> Balance/1

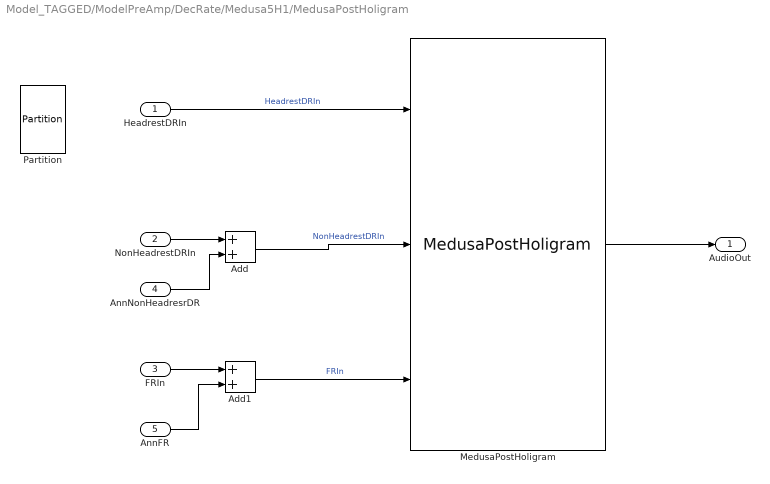
== system Model_TAGGED/ModelPreAmp/DecRate/Medusa5H1/MedusaPostHoligram ==
  HeadrestDRIn : Inport
  NonHeadrestDRIn : Inport  Port=2
  FRIn : Inport  Port=3
  AnnNonHeadresrDR : Inport  Port=4
  AnnFR : Inport  Port=5
  Add : Sum
  Add1 : Sum
  MedusaPostHoligram : medusa5h1_stereo/MedusaPostHoligram  config=Config.MedusaConfig
  Partition : FeaturePath/Partition  PartitionNumber=1  TriggerInit=[-100 66 -55 134]
      settings: SourceProductName=Bose Talaria
  AudioOut : Outport
  wires:
  HeadrestDRIn/1 -> MedusaPostHoligram/1  "HeadrestDRIn"
  NonHeadrestDRIn/1 -> Add/1
  AnnNonHeadresrDR/1 -> Add/2
  Add/1 -> MedusaPostHoligram/2  "NonHeadrestDRIn"
  FRIn/1 -> Add1/1
  Add1/1 -> MedusaPostHoligram/3  "FRIn"
  AnnFR/1 -> Add1/2
  MedusaPostHoligram/1 -> AudioOut/1

== system Model_TAGGED/ModelPreAmp/DecRate/Medusa5H1/NearWiggleFilters ==
  AnnEnable : Inport
  AudioIn : Inport  Port=2
  NEAR : Subsystem  Variant=on  VariantControl=Variant1
  Partition : FeaturePath/Partition  PartitionNumber=13  TriggerInit=[255 -129 300 -61]
      settings: SourceProductName=Bose Talaria
  Out1 : Outport
  wires:
  AnnEnable/1 -> NEAR/2(AnnEnable)
  AudioIn/1 -> NEAR/1(AudioIn)
  NEAR/1(AudioOut) -> Out1/1

== system Model_TAGGED/ModelPreAmp/DecRate/Medusa5H1/SleepingBeauty ==
  DR_In : Inport
  FR_In : Inport  Port=2
  Partition : FeaturePath/Partition  PartitionNumber=9  TriggerInit=[290 -9 335 59]
      settings: SourceProductName=Bose Talaria
  SleepingBeauty : Subsystem  Variant=on  VariantControl=Choice
  DRHeadrestComps : Outport
  SleepBeautyOut : Outport  Port=2
  FRSpkr : Outport  Port=3
  FadeGains : Outport  Port=4
  wires:
  SleepingBeauty/1(DRHeadrestComps) -> DRHeadrestComps/1  "DRHeadrestComps"
  FR_In/1 -> SleepingBeauty/2(FR)
  SleepingBeauty/4(FadeGains) -> FadeGains/1  "FadeGains"
  DR_In/1 -> SleepingBeauty/1(DR)
  SleepingBeauty/2(DRNonHeadrestSpkr) -> SleepBeautyOut/1  "SleepBeautyOut"
  SleepingBeauty/3(FRSpkr) -> FRSpkr/1  "FRSpkr"

== system Model_TAGGED/ModelPreAmp/DecRate/Medusa5H1/NearWiggleFilters/NEAR ==
  AudioIn : Inport
  AnnEnable : Inport  Port=2
  NearOff : Subsystem  VariantControl=0 == Config.NearEnable
  NearOn : Subsystem  VariantControl=0 ~= Config.NearEnable
  AudioOut : Outport

== system Model_TAGGED/ModelPreAmp/DecRate/Medusa5H1/SleepingBeauty/SleepingBeauty ==
  DR : Inport
  FR : Inport  Port=2
  Bypass : Subsystem  TreatAsAtomicUnit=on  VariantControl=Config.SleepingBeautyEnabled == 0
      settings: RTWSystemCode=Nonreusable function  RTWFcnNameOpts=Use subsystem name  RTWFileNameOpts=Use subsystem name
  Enabled : Subsystem  TreatAsAtomicUnit=on  VariantControl=(default)
      settings: RTWSystemCode=Nonreusable function  RTWFcnNameOpts=Use subsystem name  RTWFileNameOpts=Use subsystem name
  DRHeadrestComps : Outport
  DRNonHeadrestSpkr : Outport  Port=2
  FRSpkr : Outport  Port=3
  FadeGains : Outport  Port=4

== system Model_TAGGED/ModelPreAmp/DecRate/Medusa5H1/NearWiggleFilters/NEAR/NearOff ==
  AudioIn : Inport
  AnnEnable : Inport  Port=2
  Terminator1 : Terminator
  AudioOut : Outport
  wires:
  AudioIn/1 -> AudioOut/1
  AnnEnable/1 -> Terminator1/1

== system Model_TAGGED/ModelPreAmp/DecRate/Medusa5H1/NearWiggleFilters/NEAR/NearOn ==
  AudioIn : Inport
  AnnEnable : Inport  Port=2
  WiggleFilter : WiggleFilterLib/WiggleFilter  Config=Config.NearWiggleFilter
  AudioOut : Outport
  wires:
  AnnEnable/1 -> WiggleFilter/2
  AudioIn/1 -> WiggleFilter/1
  WiggleFilter/1 -> AudioOut/1

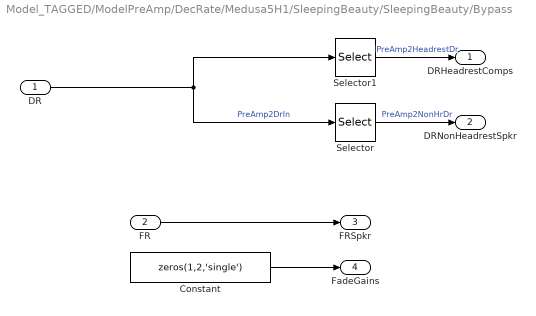
== system Model_TAGGED/ModelPreAmp/DecRate/Medusa5H1/SleepingBeauty/SleepingBeauty/Bypass ==
  DR : Inport
  FR : Inport  Port=2
  Constant : Constant  Value=zeros(1,2,'single')
  Selector : Selector  NumberOfDimensions=2  InputPortWidth=3  IndexOptions=Select all,Index vector (dialog)  Indices=[1 3],1:MedusaConfig.numNonHeadrest  OutputSizes=1,1
  Selector1 : Selector  NumberOfDimensions=2  InputPortWidth=3  IndexOptions=Select all,Index vector (dialog)  Indices=[1 3],MedusaConfig.numNonHeadrest+1:MedusaConfig.numDRChan  OutputSizes=1,1
  DRHeadrestComps : Outport
  DRNonHeadrestSpkr : Outport  Port=2
  FRSpkr : Outport  Port=3
  FadeGains : Outport  Port=4
  wires:
  Selector1/1 -> DRHeadrestComps/1  "PreAmp2HeadrestDr"
  Selector/1 -> DRNonHeadrestSpkr/1  "PreAmp2NonHrDr"
  Constant/1 -> FadeGains/1
  FR/1 -> FRSpkr/1
  DR/1 -> Selector/1, Selector1/1  "PreAmp2DrIn"

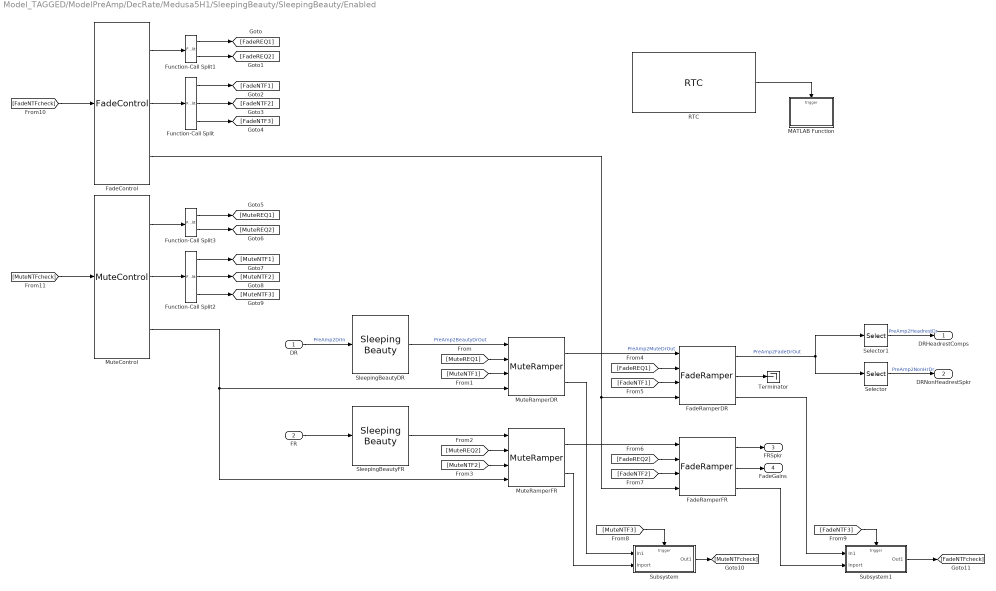
== system Model_TAGGED/ModelPreAmp/DecRate/Medusa5H1/SleepingBeauty/SleepingBeauty/Enabled ==
  DR : Inport
  FR : Inport  Port=2
  FadeControl : FadeControl/FadeControl  BankNumber=0  MaskIndexOffset=128  MaskBoostDisable=off  MaskSilentExtreme=on
  FadeRamperDR : FadeRamper/FadeRamper  MaskFeatureName=FadeRamperDR  MaskChanRampMap=ones(1,30)  MaskEnableGainPort=on
  FadeRamperFR : FadeRamper/FadeRamper  MaskFeatureName=FadeRamperFR  MaskChanRampMap=ones(1,22)  MaskEnableGainPort=on
  Function-Call Split : FunctionCallSplit  IconShape=distinctive  NumOutputPorts=3  OutputPortLayout=default
  Function-Call Split1 : FunctionCallSplit  IconShape=distinctive  NumOutputPorts=2  OutputPortLayout=default
  Function-Call Split2 : FunctionCallSplit  IconShape=distinctive  NumOutputPorts=3  OutputPortLayout=default
  Function-Call Split3 : FunctionCallSplit  IconShape=distinctive  NumOutputPorts=2  OutputPortLayout=default
  MATLAB Function : MATLAB Function  TreatAsAtomicUnit=on
  MuteControl : MuteControl/MuteControl
  MuteRamperDR : MuteRamper/MuteRamper  initial_mute_state=0  samplesPerFrame=8  MaskFeatureName=MuteDR
  MuteRamperFR : MuteRamper/MuteRamper  initial_mute_state=0  samplesPerFrame=32  MaskFeatureName=MuteFR
  RTC : RTC/RTC  REQ_Priority=RTC_Mask.NormalPriority  RequestAtInit=off  EnableRequest=on  REQElemType1=uint32  REQElemWidth1=1  REQElemInitial1=[]  REQElemType2=uint32  REQElemWidth2=1  REQElemInitial2=[]  REQElemType3=uint32  REQElemWidth3=1  REQElemInitial3=[]  REQElemType4=uint32  REQElemWidth4=1  REQElemInitial4=[]  REQElemType5=uint32  REQElemWidth5=1  REQElemInitial5=[]  REQElemType6=uint32  REQElemWidth6=1  REQElemInitial6=[]  REQElemType7=uint32  REQElemWidth7=1  REQElemInitial7=[]  REQElemType8=uint32  REQElemWidth8=1  REQElemInitial8=[]  REQElemType9=uint32  REQElemWidth9=1  REQElemInitial9=[]  REQElemType10=uint32  REQElemWidth10=1  REQElemInitial10=[]  EnableResponse=on  EnableRSP_StatusIn=off  RSPElemType1=uint32  RSPElemWidth1=1  RSPElemType2=uint32  RSPElemWidth2=1  RSPElemType3=uint32  RSPElemWidth3=1  RSPElemType4=uint32  RSPElemWidth4=1  RSPElemType5=uint32  RSPElemWidth5=1  RSPElemType6=uint32  RSPElemWidth6=1  RSPElemType7=uint32  RSPElemWidth7=1  RSPElemType8=uint32  RSPElemWidth8=1  RSPElemType9=uint32  RSPElemWidth9=1  RSPElemType10=uint32  RSPElemWidth10=1  EnableNotification=off  EnableNTF_PrepTrig=off  NTFElemType1=uint32  NTFElemWidth1=1  NTFElemType2=uint32  NTFElemWidth2=1  NTFElemType3=uint32  NTFElemWidth3=1  NTFElemType4=uint32  NTFElemWidth4=1  NTFElemType5=uint32  NTFElemWidth5=1  NTFElemType6=uint32  NTFElemWidth6=1  NTFElemType7=uint32  NTFElemWidth7=1  NTFElemType8=uint32  NTFElemWidth8=1  NTFElemType9=uint32  NTFElemWidth9=1  NTFElemType10=uint32  NTFElemWidth10=1  MaskMessageName=ResetSleepingBeauty
      settings: SourceProductName=Bose Talaria
  Selector : Selector  NumberOfDimensions=2  InputPortWidth=3  IndexOptions=Select all,Index vector (dialog)  Indices=[1 3],1:MedusaConfig.numNonHeadrest  OutputSizes=1,1
  Selector1 : Selector  NumberOfDimensions=2  InputPortWidth=3  IndexOptions=Select all,Index vector (dialog)  Indices=[1 3],MedusaConfig.numNonHeadrest+1:MedusaConfig.numDRChan  OutputSizes=1,1
  SleepingBeautyDR : SleepingBeauty/Sleeping Beauty  MaskFeatureName=SleepingBeautyDR  MaskChanRampMap=ones(1,30)  MaskOffset=128  MaskSilentExtremeMutesBass=off
  SleepingBeautyFR : SleepingBeauty/Sleeping Beauty  MaskFeatureName=SleepingBeautyFR  MaskChanRampMap=ones(1,22)  MaskOffset=128  MaskSilentExtremeMutesBass=off
  Subsystem : Subsystem
  Subsystem1 : Subsystem
  Terminator : Terminator
  DRHeadrestComps : Outport
  DRNonHeadrestSpkr : Outport  Port=2
  FRSpkr : Outport  Port=3
  FadeGains : Outport  Port=4
  wires:
  Function-Call Split2/3 -> [MuteNTF3]
  [FadeNTF1] -> FadeRamperDR/3
  FR/1 -> SleepingBeautyFR/1
  Function-Call Split2/2 -> [MuteNTF2]
  Function-Call Split3/2 -> [MuteREQ2]
  MuteControl/2 -> Function-Call Split2/1
  [FadeREQ2] -> FadeRamperFR/2
  Function-Call Split1/2 -> [FadeREQ2]
  FadeControl/2 -> Function-Call Split/1
  [FadeNTF3] -> Subsystem1/Trigger
  Function-Call Split1/1 -> [FadeREQ1]
  [MuteREQ2] -> MuteRamperFR/2
  [MuteNTF3] -> Subsystem/Trigger
  [MuteNTF1] -> MuteRamperDR/3
  [FadeNTF2] -> FadeRamperFR/3
  FadeControl/1 -> Function-Call Split1/1
  [FadeNTFcheck] -> FadeControl/1
  MuteRamperDR/1 -> FadeRamperDR/1  "PreAmp2MuteDrOut"
  [MuteREQ1] -> MuteRamperDR/2
  Function-Call Split2/1 -> [MuteNTF1]
  Function-Call Split3/1 -> [MuteREQ1]
  SleepingBeautyDR/1 -> MuteRamperDR/1  "PreAmp2BeautyDrOut"
  RTC/1 -> MATLAB Function/Trigger
  FadeRamperDR/2 -> Terminator/1
  Selector1/1 -> DRHeadrestComps/1  "PreAmp2HeadrestDr"
  MuteRamperFR/2 -> Subsystem/2(Inport)
  Selector/1 -> DRNonHeadrestSpkr/1  "PreAmp2NonHrDr"
  Subsystem/1(Out1) -> [MuteNTFcheck]
  [MuteNTFcheck] -> MuteControl/1
  [FadeREQ1] -> FadeRamperDR/2
  [MuteNTF2] -> MuteRamperFR/3
  MuteControl/1 -> Function-Call Split3/1
  Function-Call Split/2 -> [FadeNTF2]
  FadeRamperDR/3 -> Subsystem1/1(In1)
  FadeRamperFR/2 -> FadeGains/1
  Subsystem1/1(Out1) -> [FadeNTFcheck]
  FadeRamperFR/3 -> Subsystem1/2(Inport)
  SleepingBeautyFR/1 -> MuteRamperFR/1
  DR/1 -> SleepingBeautyDR/1  "PreAmp2DrIn"
  MuteRamperDR/2 -> Subsystem/1(In1)
  FadeRamperFR/1 -> FRSpkr/1
  Function-Call Split/3 -> [FadeNTF3]
  FadeRamperDR/1 -> Selector1/1, Selector/1  "PreAmp2FadeDrOut"
  MuteControl/3 -> MuteRamperFR/4, MuteRamperDR/4
  Function-Call Split/1 -> [FadeNTF1]
  MuteRamperFR/1 -> FadeRamperFR/1
  FadeControl/3 -> FadeRamperFR/4, FadeRamperDR/4

== system Model_TAGGED/ModelPreAmp/DecRate/Medusa5H1/SleepingBeauty/SleepingBeauty/Enabled/Subsystem ==
  In1 : Inport
  Inport : Inport  Port=2
  Trigger : TriggerPort  TriggerType=function-call  VariantControl=Variant  PortDimensions=1
  AND : Logic  IconShape=distinctive  AllPortsSameDT=off  OutDataTypeStr=boolean
  Out1 : Outport
  wires:
  In1/1 -> AND/1
  AND/1 -> Out1/1
  Inport/1 -> AND/2

== system Model_TAGGED/ModelPreAmp/DecRate/Medusa5H1/SleepingBeauty/SleepingBeauty/Enabled/Subsystem1 ==
  In1 : Inport
  Inport : Inport  Port=2
  Trigger : TriggerPort  TriggerType=function-call  VariantControl=Variant  PortDimensions=1
  AND : Logic  IconShape=distinctive  AllPortsSameDT=off  OutDataTypeStr=boolean
  Out1 : Outport
  wires:
  In1/1 -> AND/1
  AND/1 -> Out1/1
  Inport/1 -> AND/2

== matlab function Model_TAGGED/NEAR/MATLAB Function ==
  data: u input; y output
function y = fcn(u)

y = u;
